simulink model "stereo_ibvs_core_backup_20260724_010315"  (R2025b)
settings: Solver=FixedStepDiscrete  StartTime=0.0  StopTime=10  FixedStep=cfg.Ts  RelTol=1e-3
InitFcn:
  | modelPath = get_param(bdroot,'FileName');
  |                                                                                       simulinkPath = fileparts(fileparts(modelPath));
  |                                                                                       configPath = fullfile(simulinkPath,'config','stereo_ibvs_config.m');
  |                                                                                       if ~isfile(configPath), error('StereoIBVS:ConfigNotFound','找不到配置文件：%s',configPath); end
  |                                                                                       run(configPath);
undefined symbols (not defined in the file): cfg
(part 4 of 4)

== matlab function stereo_ibvs_core_backup_20260724_010315/01_Input_Validity/Input Validity ==
  data: qRaw input; q output; visionFeatureRaw input; focalLengthMeasuredMmRaw input; visionMeasurementNewRaw input; focalLengthIsNewRaw input; controllerEnableRaw input; resetRaw input; qInitial input; focalLength0Mm input; visionFeature output; focalLengthMeasuredMm output; visionMeasurementNewSafe output; focalLengthIsNewSafe output; controllerEnableSafe output; resetSafe output; inputDataValid output
function [ ...
    q, ...
    visionFeature, ...
    focalLengthMeasuredMm, ...
    visionMeasurementNewSafe, ...
    focalLengthIsNewSafe, ...
    controllerEnableSafe, ...
    resetSafe, ...
    inputDataValid] = fcn( ...
    qRaw, ...
    visionFeatureRaw, ...
    focalLengthMeasuredMmRaw, ...
    visionMeasurementNewRaw, ...
    focalLengthIsNewRaw, ...
    controllerEnableRaw, ...
    resetRaw, ...
    qInitial, ...
    focalLength0Mm)
%#codegen
% 检查并保存最近一次合法的关节、视觉和焦距输入。
% Core内部焦距统一使用mm。

persistent lastQ
persistent lastVisionFeature
persistent lastFocalLengthMeasuredMm

initialQ = reshape(qInitial,7,1);
initialFocalLengthMm = reshape(focalLength0Mm,2,1);

if isempty(lastQ)
    lastQ = initialQ;
    lastVisionFeature = zeros(8,1);
    lastFocalLengthMeasuredMm = initialFocalLengthMm;
end

qCandidate = reshape(qRaw,7,1);
visionCandidate = reshape(visionFeatureRaw,8,1);
focalCandidate = reshape(focalLengthMeasuredMmRaw,2,1);

qValid = all(isfinite(qCandidate));
visionValid = all(isfinite(visionCandidate));
focalValid = all(isfinite(focalCandidate));
visionNewValid = isfinite(visionMeasurementNewRaw);
focalNewValid = isfinite(focalLengthIsNewRaw);
enableValid = isfinite(controllerEnableRaw);
resetValid = isfinite(resetRaw);

visionMeasurementNewSafe = double( ...
    visionNewValid && visionMeasurementNewRaw > 0.5);

focalLengthIsNewSafe = double( ...
    focalNewValid && focalLengthIsNewRaw > 0.5);

if qValid
    lastQ = qCandidate;
end

if visionValid && visionMeasurementNewSafe > 0.5
    lastVisionFeature = visionCandidate;
end

if focalValid && focalLengthIsNewSafe > 0.5
    lastFocalLengthMeasuredMm = focalCandidate;
end

q = lastQ;
visionFeature = lastVisionFeature;
focalLengthMeasuredMm = lastFocalLengthMeasuredMm;

inputDataValid = double( ...
    qValid && ...
    visionValid && ...
    focalValid && ...
    visionNewValid && ...
    focalNewValid && ...
    enableValid && ...
    resetValid);

controllerEnableSafe = double( ...
    inputDataValid > 0.5 && ...
    controllerEnableRaw > 0.5);

if resetValid
    resetSafe = double(resetRaw > 0.5);
else
    resetSafe = 0;
end

if resetSafe > 0.5
    lastQ = initialQ;
    lastVisionFeature = zeros(8,1);
    lastFocalLengthMeasuredMm = initialFocalLengthMm;

    q = lastQ;
    visionFeature = lastVisionFeature;
    focalLengthMeasuredMm = lastFocalLengthMeasuredMm;
    visionMeasurementNewSafe = 0;
    focalLengthIsNewSafe = 0;
    controllerEnableSafe = 0;
end
end
